simulink library "ammclib_bam_s32k14x"  (Simulink 9.0)
settings: Solver=ode45  StartTime=0.0  StopTime=10.0  RelTol=1e-3
undefined symbols (not defined in the file): f16A1, f16A2, f16B0, f16B1, f16B2, f16C1, f16CC1, f16CC1sc, f16CC1sc_D, f16CC1sc_Q, f16CC1scD, f16CC1scQ, f16CC2, f16CC2sc, f16CC2sc_D, f16CC2sc_Q, f16CC2scD, f16CC2scQ, f16DerivGain, f16EGain, f16FiltCoef, f16HystOff, f16HystOn, f16IGain, f16IntegGain, f16IntegGainFW, f16IntegGainQ, f16Kd, f16Kq, f16Limit, f16LowerLim, f16LowerLimit_D, f16LowerLimit_Q, f16ModIndex, f16OutValOff, f16OutValOn, f16PropGain, f16PropGainFW, f16PropGainQ, f16RampDown, f16RampUp, f16UGain, f16UpperLim, f16UpperLimit, f16UpperLimit_D, f16UpperLimit_Q, f16WIGain, f32A1, f32A2, f32B0, f32B1, f32B2, f32C1, f32CC1, f32CC1sc, f32CC1sc_D, f32CC1sc_Q, f32CC1scD, f32CC1scQ, f32CC2 ... (+122)
(part 6 of 11)

== system ammclib_bam_s32k14x/GFLIB/bam_f16/GFLIB_ControllerPIDpAW_F16 ==
  note: ---------------------------------------------------------------------------------------------------------------------------------------------------------------------------------------------------
  f16InErr : Inport
  f16UpperLimit : Inport  Port=2
  f16LowerLimit : Inport  Port=3
  GFLIB_ControllerPIDpAW_SF : S-Function  FunctionName=GFLIB_ControllerPIDpAW_SF_F16  Parameters=f16PropGain,s16PropGainShift,f16IntegGain,s16IntegGainShift,f16DerivGain,s16DerivGainShift,f16FiltCoef  SFunctionDeploymentMode=off  EnableBusSupport=off
  Unit_Delay_f16DerivPartK_1 : Delay  DelayLength=1  InitialCondition=0
  Unit_Delay_f16InK_1 : Delay  DelayLength=1  InitialCondition=0
  Unit_Delay_f32IntegPartK_1 : Delay  DelayLength=1  InitialCondition=0
  copyright : Subsystem
      mask Display: text(10,90,'FILE:');text(10,75,'DESRIPTION:');text(10,60,'COPYRIGHT:');text(10,45,'VERSION:');text(10,30,'DATE:')
  copyright2 : Subsystem
      mask Display: text(10,90,'GFLIB_ControllerPIDpAW_BAM_F16.mdl');text(10,75,'Parallel form of a standard PID controller with implemented anti-windup.');text(10,60,'NXP');text(10,45,'0.1');text(10,30,'21-Nov-2018');
  logo : Subsystem
      mask Display: image(imread('logo.jpg'))
  f16Out : Outport
  u16LimitFlag : Outport  Port=2
  wires:
  f16InErr/1 -> GFLIB_ControllerPIDpAW_SF/1
  f16UpperLimit/1 -> GFLIB_ControllerPIDpAW_SF/2
  f16LowerLimit/1 -> GFLIB_ControllerPIDpAW_SF/3
  Unit_Delay_f16InK_1/1 -> GFLIB_ControllerPIDpAW_SF/4
  Unit_Delay_f32IntegPartK_1/1 -> GFLIB_ControllerPIDpAW_SF/5
  Unit_Delay_f16DerivPartK_1/1 -> GFLIB_ControllerPIDpAW_SF/6
  GFLIB_ControllerPIDpAW_SF/1 -> f16Out/1
  GFLIB_ControllerPIDpAW_SF/2 -> u16LimitFlag/1
  GFLIB_ControllerPIDpAW_SF/3 -> Unit_Delay_f16InK_1/1
  GFLIB_ControllerPIDpAW_SF/4 -> Unit_Delay_f32IntegPartK_1/1
  GFLIB_ControllerPIDpAW_SF/5 -> Unit_Delay_f16DerivPartK_1/1

== system ammclib_bam_s32k14x/GFLIB/bam_f16/GFLIB_ControllerPIpAW_F16 ==
  note: ---------------------------------------------------------------------------------------------------------------------------------------------------------------------------------------------------
  f16InErr : Inport
  f16UpperLimit : Inport  Port=2
  f16LowerLimit : Inport  Port=3
  GFLIB_ControllerPIpAW_SF : S-Function  FunctionName=GFLIB_ControllerPIpAW_SF_F16  Parameters=f16PropGain,s16PropGainShift,f16IntegGain,s16IntegGainShift  SFunctionDeploymentMode=off  EnableBusSupport=off
  Unit_Delay_f16InK_1 : Delay  DelayLength=1  InitialCondition=0
  Unit_Delay_f32IntegPartK_1 : Delay  DelayLength=1  InitialCondition=0
  copyright : Subsystem
      mask Display: text(10,90,'FILE:');text(10,75,'DESRIPTION:');text(10,60,'COPYRIGHT:');text(10,45,'VERSION:');text(10,30,'DATE:')
  copyright2 : Subsystem
      mask Display: text(10,90,'GFLIB_ControllerPIpAW_BAM_F16.mdl');text(10,75,'Parallel form of a standard PI controller with implemented anti-windup.');text(10,60,'NXP');text(10,45,'0.1');text(10,30,'12-Jun-2015');
  logo : Subsystem
      mask Display: image(imread('logo.jpg'))
  f16Out : Outport
  u16LimitFlag : Outport  Port=2
  wires:
  GFLIB_ControllerPIpAW_SF/2 -> u16LimitFlag/1
  GFLIB_ControllerPIpAW_SF/1 -> f16Out/1
  f16LowerLimit/1 -> GFLIB_ControllerPIpAW_SF/3
  f16UpperLimit/1 -> GFLIB_ControllerPIpAW_SF/2
  f16InErr/1 -> GFLIB_ControllerPIpAW_SF/1
  Unit_Delay_f32IntegPartK_1/1 -> GFLIB_ControllerPIpAW_SF/5
  Unit_Delay_f16InK_1/1 -> GFLIB_ControllerPIpAW_SF/4
  GFLIB_ControllerPIpAW_SF/4 -> Unit_Delay_f32IntegPartK_1/1
  GFLIB_ControllerPIpAW_SF/3 -> Unit_Delay_f16InK_1/1

== system ammclib_bam_s32k14x/GFLIB/bam_f16/GFLIB_ControllerPIp_F16 ==
  note: ---------------------------------------------------------------------------------------------------------------------------------------------------------------------------------------------------
  f16InErr : Inport
  GFLIB_ControllerPIp_SF : S-Function  FunctionName=GFLIB_ControllerPIp_SF_F16  Parameters=f16PropGain,s16PropGainShift,f16IntegGain,s16IntegGainShift  SFunctionDeploymentMode=off  EnableBusSupport=off
  Unit_Delay_f32InIntegPartK_1 : UnitDelay  SampleTime=-1
  Unit_Delay_f32InK_1 : UnitDelay  SampleTime=-1
  copyright : Subsystem
      mask Display:
      | text(10,90,'FILE:');text(10,75,'DESRIPTION:')
      | text(10,60,'COPYRIGHT:')
      | text(10,45,'VERSION:')
      | text(10,30,'DATE:')
  copyright2 : Subsystem
      mask Display:
      | text(10,90,'GFLIB_ControllerPIp_BAM_F16.mdl');text(10,75,'Parallel form of a standard PI controller without implemented anti-windup.');text(10,60,'NXP')
      | text(10,45,'0.1');text(10,30,'20-Jan-2012');
  logo : Subsystem
      mask Display: image(imread('logo.jpg'))
  f16Out : Outport
  wires:
  GFLIB_ControllerPIp_SF/1 -> f16Out/1
  f16InErr/1 -> GFLIB_ControllerPIp_SF/1
  GFLIB_ControllerPIp_SF/3 -> Unit_Delay_f32InIntegPartK_1/1
  GFLIB_ControllerPIp_SF/2 -> Unit_Delay_f32InK_1/1
  Unit_Delay_f32InIntegPartK_1/1 -> GFLIB_ControllerPIp_SF/3
  Unit_Delay_f32InK_1/1 -> GFLIB_ControllerPIp_SF/2

== system ammclib_bam_s32k14x/GFLIB/bam_f16/GFLIB_ControllerPIrAW_F16 ==
  note: ---------------------------------------------------------------------------------------------------------------------------------------------------------------------------------------------------
  f16InErr : Inport
  f16UpperLimit : Inport  Port=2
  f16LowerLimit : Inport  Port=3
  GFLIB_ControllerPIrAW_SF : S-Function  FunctionName=GFLIB_ControllerPIrAW_SF_F16  Parameters=f16CC1,f16CC2,u16NShift  SFunctionDeploymentMode=off  EnableBusSupport=off
  Unit_Delay_f16InErrK1 : Delay  DelayLength=1  InitialCondition=0
  Unit_Delay_f32Acc : Delay  DelayLength=1  InitialCondition=0
  copyright : Subsystem
      mask Display: text(10,90,'FILE:');text(10,75,'DESRIPTION:');text(10,60,'COPYRIGHT:');text(10,45,'VERSION:');text(10,30,'DATE:')
  copyright2 : Subsystem
      mask Display: text(10,90,'GFLIB_ControllerPIrAW_BAM_F16.mdl');text(10,75,'Recurrent form of a standard PI controller with implemented anti-windup functionality.');text(10,60,'NXP');text(10,45,'0.1');text(10,30,'12-Jun-2015');
  logo : Subsystem
      mask Display: image(imread('logo.jpg'))
  f16Out : Outport
  wires:
  GFLIB_ControllerPIrAW_SF/3 -> Unit_Delay_f16InErrK1/1
  GFLIB_ControllerPIrAW_SF/2 -> Unit_Delay_f32Acc/1
  GFLIB_ControllerPIrAW_SF/1 -> f16Out/1
  f16LowerLimit/1 -> GFLIB_ControllerPIrAW_SF/3
  f16UpperLimit/1 -> GFLIB_ControllerPIrAW_SF/2
  f16InErr/1 -> GFLIB_ControllerPIrAW_SF/1
  Unit_Delay_f16InErrK1/1 -> GFLIB_ControllerPIrAW_SF/5
  Unit_Delay_f32Acc/1 -> GFLIB_ControllerPIrAW_SF/4

== system ammclib_bam_s32k14x/GFLIB/bam_f16/GFLIB_ControllerPIr_F16 ==
  note: ---------------------------------------------------------------------------------------------------------------------------------------------------------------------------------------------------
  f16InErr : Inport
  GFLIB_ControllerPIr_SF : S-Function  FunctionName=GFLIB_ControllerPIr_SF_F16  Parameters=f16CC1,f16CC2,u16NShift  SFunctionDeploymentMode=off  EnableBusSupport=off
  Unit_Delay_f16InErrK_1 : UnitDelay  SampleTime=-1
  Unit_Delay_f32AccIn : UnitDelay  SampleTime=-1
  copyright : Subsystem
      mask Display:
      | text(10,90,'FILE:');text(10,75,'DESRIPTION:')
      | text(10,60,'COPYRIGHT:')
      | text(10,45,'VERSION:')
      | text(10,30,'DATE:')
  copyright2 : Subsystem
      mask Display:
      | text(10,90,'GFLIB_ControllerPIr_BAM_F16.mdl');text(10,75,'Recurrent form of a standard PI controller without implemented anti-windup.');text(10,60,'NXP')
      | text(10,45,'0.1');text(10,30,'20-Jan-2012');
  logo : Subsystem
      mask Display: image(imread('logo.jpg'))
  f16Out : Outport
  wires:
  GFLIB_ControllerPIr_SF/1 -> f16Out/1
  f16InErr/1 -> GFLIB_ControllerPIr_SF/1
  GFLIB_ControllerPIr_SF/3 -> Unit_Delay_f16InErrK_1/1
  GFLIB_ControllerPIr_SF/2 -> Unit_Delay_f32AccIn/1
  Unit_Delay_f16InErrK_1/1 -> GFLIB_ControllerPIr_SF/3
  Unit_Delay_f32AccIn/1 -> GFLIB_ControllerPIr_SF/2

== system ammclib_bam_s32k14x/GFLIB/bam_f16/GFLIB_Cos_F16 ==
  note: ---------------------------------------------------------------------------------------------------------------------------------------------------------------------------------------------------
  f16In : Inport
  GFLIB_Cos_SF : S-Function  FunctionName=GFLIB_Cos_SF_F16  SFunctionDeploymentMode=off  EnableBusSupport=off
  copyright : Subsystem
      mask Display:
      | text(10,90,'FILE:');text(10,75,'DESRIPTION:')
      | text(10,60,'COPYRIGHT:')
      | text(10,45,'VERSION:')
      | text(10,30,'DATE:')
  copyright2 : Subsystem
      mask Display:
      | text(10,90,'GFLIB_Cos_BAM_F16.mdl');text(10,75,'Cosine transformation');text(10,60,'NXP')
      | text(10,45,'0.1');text(10,30,'13-Sep-2011');
  logo : Subsystem
      mask Display: image(imread('logo.jpg'))
  f16Out : Outport
  wires:
  GFLIB_Cos_SF/1 -> f16Out/1
  f16In/1 -> GFLIB_Cos_SF/1

== system ammclib_bam_s32k14x/GFLIB/bam_f16/GFLIB_Hyst_F16 ==
  note: ---------------------------------------------------------------------------------------------------------------------------------------------------------------------------------------------------
  f16In : Inport
  GFLIB_Hyst_SF_F16 : S-Function  FunctionName=GFLIB_Hyst_SF_F16  Parameters=f16HystOn,f16HystOff,f16OutValOn,f16OutValOff  SFunctionDeploymentMode=off  EnableBusSupport=off
  Unit_Delay_f16InState : UnitDelay  SampleTime=-1
  copyright : Subsystem
      mask Display:
      | text(10,90,'FILE:');text(10,75,'DESRIPTION:')
      | text(10,60,'COPYRIGHT:')
      | text(10,45,'VERSION:')
      | text(10,30,'DATE:')
  copyright2 : Subsystem
      mask Display:
      | text(10,90,'GFLIB_Hyst_BAM_F16.mdl');text(10,75,'Hysteresis function.');text(10,60,'NXP')
      | text(10,45,'0.1');text(10,30,'09-Apr-2014');
  logo : Subsystem
      mask Display: image(imread('logo.jpg'))
  f16Out : Outport
  wires:
  GFLIB_Hyst_SF_F16/1 -> f16Out/1
  f16In/1 -> GFLIB_Hyst_SF_F16/1
  Unit_Delay_f16InState/1 -> GFLIB_Hyst_SF_F16/2
  GFLIB_Hyst_SF_F16/2 -> Unit_Delay_f16InState/1

== system ammclib_bam_s32k14x/GFLIB/bam_f16/GFLIB_IntegratorTR_F16 ==
  note: ---------------------------------------------------------------------------------------------------------------------------------------------------------------------------------------------------
  f16In : Inport
  GFLIB_IntegratorTR_SF : S-Function  FunctionName=GFLIB_IntegratorTR_SF_F16  Parameters=f16C1,u16NShift  SFunctionDeploymentMode=off  EnableBusSupport=off
  Unit_Delay_f16InK_1 : UnitDelay  SampleTime=-1
  Unit_Delay_f32InAcc : UnitDelay  SampleTime=-1
  copyright : Subsystem
      mask Display:
      | text(10,90,'FILE:');text(10,75,'DESRIPTION:')
      | text(10,60,'COPYRIGHT:')
      | text(10,45,'VERSION:')
      | text(10,30,'DATE:')
  copyright2 : Subsystem
      mask Display:
      | text(10,90,'GFLIB_IntegratorTR_BAM_F16.mdl');text(10,75,'Discrete integrator transformed from linear model using Billinear (trapezoidal) transformation.');text(10,60,'NXP')
      | text(10,45,'0.1');text(10,30,'16-Jan-2012');
  logo : Subsystem
      mask Display: image(imread('logo.jpg'))
  f16Out : Outport
  wires:
  GFLIB_IntegratorTR_SF/1 -> f16Out/1
  f16In/1 -> GFLIB_IntegratorTR_SF/1
  Unit_Delay_f16InK_1/1 -> GFLIB_IntegratorTR_SF/3
  GFLIB_IntegratorTR_SF/3 -> Unit_Delay_f16InK_1/1
  Unit_Delay_f32InAcc/1 -> GFLIB_IntegratorTR_SF/2
  GFLIB_IntegratorTR_SF/2 -> Unit_Delay_f32InAcc/1

== system ammclib_bam_s32k14x/GFLIB/bam_f16/GFLIB_Limit_F16 ==
  note: ---------------------------------------------------------------------------------------------------------------------------------------------------------------------------------------------------
  f16In : Inport
  GFLIB_Limit_SF_F16 : S-Function  FunctionName=GFLIB_Limit_SF_F16  Parameters=f16UpperLimit,f16LowerLim  SFunctionDeploymentMode=off  EnableBusSupport=off
  copyright : Subsystem
      mask Display:
      | text(10,90,'FILE:');text(10,75,'DESRIPTION:')
      | text(10,60,'COPYRIGHT:')
      | text(10,45,'VERSION:')
      | text(10,30,'DATE:')
      | text(10,15,'AUTHOR:')
  copyright2 : Subsystem
      mask Display:
      | text(10,90,'GFLIB_Limit_BAM_F16.mdl');text(10,75,'Limit function');text(10,60,'NXP')
      | text(10,45,'0.1');text(10,30,'03-Jul-2011');text(10,15,'');
  logo : Subsystem
      mask Display: image(imread('logo.jpg'))
  f16Out : Outport
  wires:
  GFLIB_Limit_SF_F16/1 -> f16Out/1
  f16In/1 -> GFLIB_Limit_SF_F16/1

== system ammclib_bam_s32k14x/GFLIB/bam_f16/GFLIB_LowerLimit_F16 ==
  note: ---------------------------------------------------------------------------------------------------------------------------------------------------------------------------------------------------
  f16In : Inport
  GFLIB_LowerLimit_SF_F16 : S-Function  FunctionName=GFLIB_LowerLimit_SF_F16  Parameters=f16LowerLim  SFunctionDeploymentMode=off  EnableBusSupport=off
  copyright : Subsystem
      mask Display:
      | text(10,90,'FILE:');text(10,75,'DESRIPTION:')
      | text(10,60,'COPYRIGHT:')
      | text(10,45,'VERSION:')
      | text(10,30,'DATE:')
  copyright2 : Subsystem
      mask Display:
      | text(10,90,'GFLIB_LowerLimit_BAM_F16.mdl');text(10,75,'Lower limit function.');text(10,60,'Freescale')
      | text(10,45,'0.1');text(10,30,'13-Sep-2011');
  logo : Subsystem
      mask Display: image(imread('logo.jpg'))
  f16Out : Outport
  wires:
  GFLIB_LowerLimit_SF_F16/1 -> f16Out/1
  f16In/1 -> GFLIB_LowerLimit_SF_F16/1

== system ammclib_bam_s32k14x/GFLIB/bam_f16/GFLIB_Lut1D_F16 ==
  note: ---------------------------------------------------------------------------------------------------------------------------------------------------------------------------------------------------
  f16In : Inport
  GFLIB_Lut1D_SF : S-Function  FunctionName=GFLIB_Lut1D_SF_F16  Parameters=u16ShamOffset,pf16Table,s16MidIdx  SFunctionDeploymentMode=off  EnableBusSupport=off
  copyright : Subsystem
      mask Display:
      | text(10,90,'FILE:');text(10,75,'DESRIPTION:')
      | text(10,60,'COPYRIGHT:')
      | text(10,45,'VERSION:')
      | text(10,30,'DATE:')
  copyright2 : Subsystem
      mask Display:
      | text(10,90,'GFLIB_Lut1D_BAM_F16.mdl');text(10,75,'One dimensional Look-up table function');text(10,60,'NXP')
      | text(10,45,'0.1');text(10,30,'17-Jun-2013');
  logo : Subsystem
      mask Display: image(imread('logo.jpg'))
  f16Out : Outport
  wires:
  GFLIB_Lut1D_SF/1 -> f16Out/1
  f16In/1 -> GFLIB_Lut1D_SF/1

== system ammclib_bam_s32k14x/GFLIB/bam_f16/GFLIB_Lut2D_F16 ==
  note: ---------------------------------------------------------------------------------------------------------------------------------------------------------------------------------------------------
  f16In1 : Inport
  f16In2 : Inport  Port=2
  GFLIB_Lut2D_SF : S-Function  FunctionName=GFLIB_Lut2D_SF_F16  Parameters=u16ShamOffset1,u16ShamOffset2,pf16Table,s16MidIdx  SFunctionDeploymentMode=off  EnableBusSupport=off
  copyright : Subsystem
      mask Display:
      | text(10,90,'FILE:');text(10,75,'DESRIPTION:')
      | text(10,60,'COPYRIGHT:')
      | text(10,45,'VERSION:')
      | text(10,30,'DATE:')
  copyright2 : Subsystem
      mask Display:
      | text(10,90,'GFLIB_Lut2D_BAM_F16.mdl');text(10,75,'Two dimensional Look-up table function');text(10,60,'NXP')
      | text(10,45,'0.1');text(10,30,'17-Jun-2013');
  logo : Subsystem
      mask Display: image(imread('logo.jpg'))
  f16Out : Outport
  wires:
  GFLIB_Lut2D_SF/1 -> f16Out/1
  f16In2/1 -> GFLIB_Lut2D_SF/2
  f16In1/1 -> GFLIB_Lut2D_SF/1

== system ammclib_bam_s32k14x/GFLIB/bam_f16/GFLIB_Ramp_F16 ==
  note: ---------------------------------------------------------------------------------------------------------------------------------------------------------------------------------------------------
  f16In : Inport
  GFLIB_Ramp_SF_F16 : S-Function  FunctionName=GFLIB_Ramp_SF_F16  Parameters=f16RampUp,f16RampDown  SFunctionDeploymentMode=off  EnableBusSupport=off
  Unit_Delay_f16InState : UnitDelay  SampleTime=-1
  copyright : Subsystem
      mask Display:
      | text(10,90,'FILE:');text(10,75,'DESRIPTION:')
      | text(10,60,'COPYRIGHT:')
      | text(10,45,'VERSION:')
      | text(10,30,'DATE:')
      | text(10,15,'AUTHOR:')
  copyright2 : Subsystem
      mask Display:
      | text(10,90,'GFLIB_Ramp_BAM_F16.mdl');text(10,75,'Rate of change limiter - Ramp function.');text(10,60,'NXP')
      | text(10,45,'0.1');text(10,30,'08-Apr-2014');text(10,15,'');
  logo : Subsystem
      mask Display: image(imread('logo.jpg'))
  f16Out : Outport
  wires:
  GFLIB_Ramp_SF_F16/1 -> f16Out/1
  f16In/1 -> GFLIB_Ramp_SF_F16/1
  Unit_Delay_f16InState/1 -> GFLIB_Ramp_SF_F16/2
  GFLIB_Ramp_SF_F16/2 -> Unit_Delay_f16InState/1

== system ammclib_bam_s32k14x/GFLIB/bam_f16/GFLIB_Sign_F16 ==
  note: ---------------------------------------------------------------------------------------------------------------------------------------------------------------------------------------------------
  f16In : Inport
  GFLIB_Sign_SF_F16 : S-Function  FunctionName=GFLIB_Sign_SF_F16  SFunctionDeploymentMode=off  EnableBusSupport=off
  copyright : Subsystem
      mask Display:
      | text(10,90,'FILE:');text(10,75,'DESRIPTION:')
      | text(10,60,'COPYRIGHT:')
      | text(10,45,'VERSION:')
      | text(10,30,'DATE:')
  copyright2 : Subsystem
      mask Display:
      | text(10,90,'GFLIB_Sign_BAM_F16.mdl');text(10,75,'Sign function.');text(10,60,'NXP')
      | text(10,45,'0.1');text(10,30,'26-Aug-2011');
  logo : Subsystem
      mask Display: image(imread('logo.jpg'))
  f16Out : Outport
  wires:
  GFLIB_Sign_SF_F16/1 -> f16Out/1
  f16In/1 -> GFLIB_Sign_SF_F16/1

== system ammclib_bam_s32k14x/GFLIB/bam_f16/GFLIB_SinCos_F16 ==
  note: ---------------------------------------------------------------------------------------------------------------------------------------------------------------------------------------------------
  f16In : Inport
  GFLIB_SinCos_SF : S-Function  FunctionName=GFLIB_SinCos_SF_F16  SFunctionDeploymentMode=off  EnableBusSupport=off
  copyright : Subsystem
      mask Display: text(10,90,'FILE:');text(10,75,'DESRIPTION:');text(10,60,'COPYRIGHT:');text(10,45,'VERSION:');text(10,30,'DATE:')
  copyright2 : Subsystem
      mask Display: text(10,90,'GFLIB_SinCos_BAM_F16.mdl');text(10,75,'Sine and Cosine transformation');text(10,60,'Freescale');text(10,45,'0.1');text(10,30,'27-Sep-2015');
  logo : Subsystem
      mask Display: image(imread('logo.jpg'))
  f16SinOut : Outport
  f16CosOut : Outport  Port=2
  wires:
  GFLIB_SinCos_SF/2 -> f16CosOut/1
  GFLIB_SinCos_SF/1 -> f16SinOut/1
  f16In/1 -> GFLIB_SinCos_SF/1

== system ammclib_bam_s32k14x/GFLIB/bam_f16/GFLIB_Sin_F16 ==
  note: ---------------------------------------------------------------------------------------------------------------------------------------------------------------------------------------------------
  f16In : Inport
  GFLIB_Sin_SF : S-Function  FunctionName=GFLIB_Sin_SF_F16  SFunctionDeploymentMode=off  EnableBusSupport=off
  copyright : Subsystem
      mask Display:
      | text(10,90,'FILE:');text(10,75,'DESRIPTION:')
      | text(10,60,'COPYRIGHT:')
      | text(10,45,'VERSION:')
      | text(10,30,'DATE:')
  copyright2 : Subsystem
      mask Display:
      | text(10,90,'GFLIB_Sin_BAM_F16.mdl');text(10,75,'Sine transformation');text(10,60,'NXP')
      | text(10,45,'0.1');text(10,30,'13-Sep-2011');
  logo : Subsystem
      mask Display: image(imread('logo.jpg'))
  f16Out : Outport
  wires:
  GFLIB_Sin_SF/1 -> f16Out/1
  f16In/1 -> GFLIB_Sin_SF/1

== system ammclib_bam_s32k14x/GFLIB/bam_f16/GFLIB_Sqrt_F16 ==
  note: ---------------------------------------------------------------------------------------------------------------------------------------------------------------------------------------------------
  f16In : Inport
  GFLIB_Sqrt_SF_F16 : S-Function  FunctionName=GFLIB_Sqrt_SF_F16  SFunctionDeploymentMode=off  EnableBusSupport=off
  copyright : Subsystem
      mask Display:
      | text(10,90,'FILE:');text(10,75,'DESRIPTION:')
      | text(10,60,'COPYRIGHT:')
      | text(10,45,'VERSION:')
      | text(10,30,'DATE:')
  copyright2 : Subsystem
      mask Display:
      | text(10,90,'GFLIB_Sqrt_BAM_F16.mdl');text(10,75,'Square root approximation.');text(10,60,'Freescale')
      | text(10,45,'0.1');text(10,30,'12-Sep-2011');
  logo : Subsystem
      mask Display: image(imread('logo.jpg'))
  f16Out : Outport
  wires:
  GFLIB_Sqrt_SF_F16/1 -> f16Out/1
  f16In/1 -> GFLIB_Sqrt_SF_F16/1

== system ammclib_bam_s32k14x/GFLIB/bam_f16/GFLIB_Tan_F16 ==
  note: ---------------------------------------------------------------------------------------------------------------------------------------------------------------------------------------------------
  f16In : Inport
  GFLIB_Tan_SF : S-Function  FunctionName=GFLIB_Tan_SF_F16  SFunctionDeploymentMode=off  EnableBusSupport=off
  copyright : Subsystem
      mask Display:
      | text(10,90,'FILE:');text(10,75,'DESRIPTION:')
      | text(10,60,'COPYRIGHT:')
      | text(10,45,'VERSION:')
      | text(10,30,'DATE:')
  copyright2 : Subsystem
      mask Display:
      | text(10,90,'GFLIB_Tan_BAM_F16.mdl');text(10,75,'Tangent transformation');text(10,60,'NXP')
      | text(10,45,'0.1');text(10,30,'13-Sep-2011');
  logo : Subsystem
      mask Display: image(imread('logo.jpg'))
  f16Out : Outport
  wires:
  GFLIB_Tan_SF/1 -> f16Out/1
  f16In/1 -> GFLIB_Tan_SF/1

== system ammclib_bam_s32k14x/GFLIB/bam_f16/GFLIB_UpperLimit_F16 ==
  note: ---------------------------------------------------------------------------------------------------------------------------------------------------------------------------------------------------
  f16In : Inport
  GFLIB_UpperLimit_SF_F16 : S-Function  FunctionName=GFLIB_UpperLimit_SF_F16  Parameters=f16UpperLim  SFunctionDeploymentMode=off  EnableBusSupport=off
  copyright : Subsystem
      mask Display:
      | text(10,90,'FILE:');text(10,75,'DESRIPTION:')
      | text(10,60,'COPYRIGHT:')
      | text(10,45,'VERSION:')
      | text(10,30,'DATE:')
  copyright2 : Subsystem
      mask Display:
      | text(10,90,'GFLIB_UpperLimit_BAM_F16.mdl');text(10,75,'Upper limit function.');text(10,60,'Freescale')
      | text(10,45,'0.1');text(10,30,'13-Sep-2011');
  logo : Subsystem
      mask Display: image(imread('logo.jpg'))
  f16Out : Outport
  wires:
  GFLIB_UpperLimit_SF_F16/1 -> f16Out/1
  f16In/1 -> GFLIB_UpperLimit_SF_F16/1

== system ammclib_bam_s32k14x/GFLIB/bam_f16/GFLIB_VMin_F16 ==
  note: ---------------------------------------------------------------------------------------------------------------------------------------------------------------------------------------------------
  InputVector : Inport
  GFLIB_VMin_SF : S-Function  FunctionName=GFLIB_VMin_SF_F16  Parameters=N  SFunctionDeploymentMode=off  EnableBusSupport=off
  Gain : Gain  Gain=[eye(N) zeros(N,256-N)]'  Multiplication=Matrix(K*u)  OutDataTypeStr=int16
  copyright : Subsystem
      mask Display: text(10,90,'FILE:');text(10,75,'DESRIPTION:');text(10,60,'COPYRIGHT:');text(10,45,'VERSION:');text(10,30,'DATE:')
  copyright2 : Subsystem
      mask Display: text(10,90,'GFLIB_VMin_BAM_F16.mdl');text(10,75,'Vector minimum');text(10,60,'NXP');text(10,45,'1.0');text(10,30,'18-Jan-2018');
  logo : Subsystem
      mask Display: image(imread('logo.jpg'))
  IndexOfMinimum : Outport
  wires:
  InputVector/1 -> Gain/1
  GFLIB_VMin_SF/1 -> IndexOfMinimum/1
  Gain/1 -> GFLIB_VMin_SF/1

== system ammclib_bam_s32k14x/GFLIB/bam_f16/GFLIB_VectorLimit_F16 ==
  note: ---------------------------------------------------------------------------------------------------------------------------------------------------------------------------------------------------
  f16InVec1 : Inport
  f16InVec2 : Inport  Port=2
  GFLIB_VectorLimit_SF_F16 : S-Function  FunctionName=GFLIB_VectorLimit_SF_F16  Parameters=f16Limit  SFunctionDeploymentMode=off  EnableBusSupport=off
  copyright : Subsystem
      mask Display:
      | text(10,90,'FILE:');text(10,75,'DESRIPTION:')
      | text(10,60,'COPYRIGHT:')
      | text(10,45,'VERSION:')
      | text(10,30,'DATE:')
      | text(10,15,'AUTHOR:')
  copyright2 : Subsystem
      mask Display:
      | text(10,90,'GFLIB_VectorLimit_BAM_F16.mdl');text(10,75,'Vector limit function');text(10,60,'Freescale')
      | text(10,45,'0.1');text(10,30,'15-Sep-2011');text(10,15,'');
  logo : Subsystem
      mask Display: image(imread('logo.jpg'))
  f16OutVec1 : Outport
  f16OutVec2 : Outport  Port=2
  bFlag : Outport  Port=3
  wires:
  GFLIB_VectorLimit_SF_F16/3 -> bFlag/1
  GFLIB_VectorLimit_SF_F16/2 -> f16OutVec2/1
  f16InVec2/1 -> GFLIB_VectorLimit_SF_F16/2
  GFLIB_VectorLimit_SF_F16/1 -> f16OutVec1/1
  f16InVec1/1 -> GFLIB_VectorLimit_SF_F16/1

== system ammclib_bam_s32k14x/GFLIB/bam_f32/GFLIB_Acos_F32 ==
  note: ---------------------------------------------------------------------------------------------------------------------------------------------------------------------------------------------------
  f32In : Inport
  GFLIB_Acos_SF : S-Function  FunctionName=GFLIB_Acos_SF_F32  SFunctionDeploymentMode=off  EnableBusSupport=off
  copyright : Subsystem
      mask Display:
      | text(10,90,'FILE:');text(10,75,'DESRIPTION:')
      | text(10,60,'COPYRIGHT:')
      | text(10,45,'VERSION:')
      | text(10,30,'DATE:')
  copyright2 : Subsystem
      mask Display:
      | text(10,90,'GFLIB_Acos_BAM_F32.mdl');text(10,75,'Inverse cosine transformation');text(10,60,'Freescale')
      | text(10,45,'0.1');text(10,30,'31-Aug-2011');
  logo : Subsystem
      mask Display: image(imread('logo.jpg'))
  f32Out : Outport
  wires:
  GFLIB_Acos_SF/1 -> f32Out/1
  f32In/1 -> GFLIB_Acos_SF/1

== system ammclib_bam_s32k14x/GFLIB/bam_f32/GFLIB_Asin_F32 ==
  note: ---------------------------------------------------------------------------------------------------------------------------------------------------------------------------------------------------
  f32In : Inport
  GFLIB_Asin_SF : S-Function  FunctionName=GFLIB_Asin_SF_F32  SFunctionDeploymentMode=off  EnableBusSupport=off
  copyright : Subsystem
      mask Display:
      | text(10,90,'FILE:');text(10,75,'DESRIPTION:')
      | text(10,60,'COPYRIGHT:')
      | text(10,45,'VERSION:')
      | text(10,30,'DATE:')
  copyright2 : Subsystem
      mask Display:
      | text(10,90,'GFLIB_Asin_BAM_F32.mdl');text(10,75,'Inverse cosine transformation');text(10,60,'Freescale')
      | text(10,45,'0.1');text(10,30,'01-Sep-2011');
  logo : Subsystem
      mask Display: image(imread('logo.jpg'))
  f32Out : Outport
  wires:
  GFLIB_Asin_SF/1 -> f32Out/1
  f32In/1 -> GFLIB_Asin_SF/1

== system ammclib_bam_s32k14x/GFLIB/bam_f32/GFLIB_AtanYXShifted_F32 ==
  note: ---------------------------------------------------------------------------------------------------------------------------------------------------------------------------------------------------
  f32InY : Inport
  f32InX : Inport  Port=2
  GFLIB_AtanYXShifted_SF : S-Function  FunctionName=GFLIB_AtanYXShifted_SF_F32  Parameters=Ky,Kx,Ny,Nx,ThetaAdj  SFunctionDeploymentMode=off  EnableBusSupport=off
  copyright : Subsystem
      mask Display:
      | text(10,90,'FILE:');text(10,75,'DESRIPTION:')
      | text(10,60,'COPYRIGHT:')
      | text(10,45,'VERSION:')
      | text(10,30,'DATE:')
  copyright2 : Subsystem
      mask Display:
      | text(10,90,'GFLIB_AtanYXShifted_BAM_F32.mdl');text(10,75,'Shifted YX Arctangent of argument.');text(10,60,'NXP')
      | text(10,45,'0.1');text(10,30,'06-Sep-2011');
  logo : Subsystem
      mask Display: image(imread('logo.jpg'))
  f32Out : Outport
  wires:
  GFLIB_AtanYXShifted_SF/1 -> f32Out/1
  f32InX/1 -> GFLIB_AtanYXShifted_SF/2
  f32InY/1 -> GFLIB_AtanYXShifted_SF/1

== system ammclib_bam_s32k14x/GFLIB/bam_f32/GFLIB_AtanYX_F32 ==
  note: ---------------------------------------------------------------------------------------------------------------------------------------------------------------------------------------------------
  f32InY : Inport
  f32InX : Inport  Port=2
  GFLIB_AtanYX_SF : S-Function  FunctionName=GFLIB_AtanYX_SF_F32  SFunctionDeploymentMode=off  EnableBusSupport=off
  copyright : Subsystem
      mask Display:
      | text(10,90,'FILE:');text(10,75,'DESRIPTION:')
      | text(10,60,'COPYRIGHT:')
      | text(10,45,'VERSION:')
      | text(10,30,'DATE:')
  copyright2 : Subsystem
      mask Display:
      | text(10,90,'GFLIB_AtanYX_BAM_F32.mdl');text(10,75,'YX Arctangent of argument.');text(10,60,'Freescale')
      | text(10,45,'0.1');text(10,30,'05-Sep-2011');
  logo : Subsystem
      mask Display: image(imread('logo.jpg'))
  f32Out : Outport
  wires:
  GFLIB_AtanYX_SF/1 -> f32Out/1
  f32InX/1 -> GFLIB_AtanYX_SF/2
  f32InY/1 -> GFLIB_AtanYX_SF/1

== system ammclib_bam_s32k14x/GFLIB/bam_f32/GFLIB_Atan_F32 ==
  note: ---------------------------------------------------------------------------------------------------------------------------------------------------------------------------------------------------
  f32In : Inport
  GFLIB_Atan_SF : S-Function  FunctionName=GFLIB_Atan_SF_F32  SFunctionDeploymentMode=off  EnableBusSupport=off
  copyright : Subsystem
      mask Display:
      | text(10,90,'FILE:');text(10,75,'DESRIPTION:')
      | text(10,60,'COPYRIGHT:')
      | text(10,45,'VERSION:')
      | text(10,30,'DATE:')
  copyright2 : Subsystem
      mask Display:
      | text(10,90,'GFLIB_Atan_BAM_F32.mdl');text(10,75,'Inverse tangent transformation');text(10,60,'Freescale')
      | text(10,45,'0.1');text(10,30,'01-Sep-2011');
  logo : Subsystem
      mask Display: image(imread('logo.jpg'))
  f32Out : Outport
  wires:
  GFLIB_Atan_SF/1 -> f32Out/1
  f32In/1 -> GFLIB_Atan_SF/1

== system ammclib_bam_s32k14x/GFLIB/bam_f32/GFLIB_ControllerPIDpAW_F32 ==
  note: ---------------------------------------------------------------------------------------------------------------------------------------------------------------------------------------------------
  f32InErr : Inport
  f32UpperLimit : Inport  Port=2
  f32LowerLimit : Inport  Port=3
  Delay : Delay  DelayLength=1  InitialCondition=0
  Delay1 : Delay  DelayLength=1  InitialCondition=0
  Delay2 : Delay  DelayLength=1  InitialCondition=0
  GFLIB_ControllerPIDpAW_SF : S-Function  FunctionName=GFLIB_ControllerPIDpAW_SF_F32  Parameters=f32PropGain,s16PropGainShift,f32IntegGain,s16IntegGainShift,f32DerivGain,s16DerivGainShift,f32FiltCoef  SFunctionDeploymentMode=off  EnableBusSupport=off
  copyright : Subsystem
      mask Display: text(10,90,'FILE:');text(10,75,'DESRIPTION:');text(10,60,'COPYRIGHT:');text(10,45,'VERSION:');text(10,30,'DATE:')
  copyright2 : Subsystem
      mask Display: text(10,90,'GFLIB_ControllerPIDpAW_BAM_F32.mdl');text(10,75,'Parallel form of a standard PID controller with implemented anti-windup.');text(10,60,'NXP');text(10,45,'0.1');text(10,30,'21-Nov-2018');
  logo : Subsystem
      mask Display: image(imread('logo.jpg'))
  f32Out : Outport
  u16LimitFlag : Outport  Port=2
  wires:
  f32InErr/1 -> GFLIB_ControllerPIDpAW_SF/1
  f32UpperLimit/1 -> GFLIB_ControllerPIDpAW_SF/2
  f32LowerLimit/1 -> GFLIB_ControllerPIDpAW_SF/3
  Delay2/1 -> GFLIB_ControllerPIDpAW_SF/4
  Delay1/1 -> GFLIB_ControllerPIDpAW_SF/5
  Delay/1 -> GFLIB_ControllerPIDpAW_SF/6
  GFLIB_ControllerPIDpAW_SF/1 -> f32Out/1
  GFLIB_ControllerPIDpAW_SF/2 -> u16LimitFlag/1
  GFLIB_ControllerPIDpAW_SF/3 -> Delay2/1
  GFLIB_ControllerPIDpAW_SF/4 -> Delay1/1
  GFLIB_ControllerPIDpAW_SF/5 -> Delay/1

== system ammclib_bam_s32k14x/GFLIB/bam_f32/GFLIB_ControllerPIpAW_F32 ==
  note: ---------------------------------------------------------------------------------------------------------------------------------------------------------------------------------------------------
  f32InErr : Inport
  f32UpperLimit : Inport  Port=2
  f32LowerLimit : Inport  Port=3
  GFLIB_ControllerPIpAW_SF : S-Function  FunctionName=GFLIB_ControllerPIpAW_SF_F32  Parameters=f32PropGain,s16PropGainShift,f32IntegGain,s16IntegGainShift  SFunctionDeploymentMode=off  EnableBusSupport=off
  Unit_Delay_f32InK_1 : Delay  DelayLength=1  InitialCondition=0
  Unit_Delay_f32IntegPartK_1 : Delay  DelayLength=1  InitialCondition=0
  copyright : Subsystem
      mask Display: text(10,90,'FILE:');text(10,75,'DESRIPTION:');text(10,60,'COPYRIGHT:');text(10,45,'VERSION:');text(10,30,'DATE:')
  copyright2 : Subsystem
      mask Display: text(10,90,'GFLIB_ControllerPIpAW_BAM_F32.mdl');text(10,75,'Parallel form of a standard PI controller with implemented anti-windup.');text(10,60,'NXP');text(10,45,'0.1');text(10,30,'12-Jun-2015');
  logo : Subsystem
      mask Display: image(imread('logo.jpg'))
  f32Out : Outport
  u16LimitFlag : Outport  Port=2
  wires:
  GFLIB_ControllerPIpAW_SF/2 -> u16LimitFlag/1
  GFLIB_ControllerPIpAW_SF/1 -> f32Out/1
  f32LowerLimit/1 -> GFLIB_ControllerPIpAW_SF/3
  f32UpperLimit/1 -> GFLIB_ControllerPIpAW_SF/2
  f32InErr/1 -> GFLIB_ControllerPIpAW_SF/1
  Unit_Delay_f32IntegPartK_1/1 -> GFLIB_ControllerPIpAW_SF/5
  Unit_Delay_f32InK_1/1 -> GFLIB_ControllerPIpAW_SF/4
  GFLIB_ControllerPIpAW_SF/4 -> Unit_Delay_f32IntegPartK_1/1
  GFLIB_ControllerPIpAW_SF/3 -> Unit_Delay_f32InK_1/1

== system ammclib_bam_s32k14x/GFLIB/bam_f32/GFLIB_ControllerPIp_F32 ==
  note: ---------------------------------------------------------------------------------------------------------------------------------------------------------------------------------------------------
  f32InErr : Inport
  GFLIB_ControllerPIp_SF : S-Function  FunctionName=GFLIB_ControllerPIp_SF_F32  Parameters=f32PropGain,s16PropGainShift,f32IntegGain,s16IntegGainShift  SFunctionDeploymentMode=off  EnableBusSupport=off
  Unit_Delay_f32InIntegPartK_1 : UnitDelay  SampleTime=-1
  Unit_Delay_f32InK_1 : UnitDelay  SampleTime=-1
  copyright : Subsystem
      mask Display:
      | text(10,90,'FILE:');text(10,75,'DESRIPTION:')
      | text(10,60,'COPYRIGHT:')
      | text(10,45,'VERSION:')
      | text(10,30,'DATE:')
  copyright2 : Subsystem
      mask Display:
      | text(10,90,'GFLIB_ControllerPIp_BAM_F32.mdl');text(10,75,'Parallel form of a standard PI controller without implemented anti-windup.');text(10,60,'NXP')
      | text(10,45,'0.1');text(10,30,'20-Jan-2012');
  logo : Subsystem
      mask Display: image(imread('logo.jpg'))
  f32Out : Outport
  wires:
  GFLIB_ControllerPIp_SF/1 -> f32Out/1
  f32InErr/1 -> GFLIB_ControllerPIp_SF/1
  GFLIB_ControllerPIp_SF/3 -> Unit_Delay_f32InIntegPartK_1/1
  Unit_Delay_f32InIntegPartK_1/1 -> GFLIB_ControllerPIp_SF/3
  Unit_Delay_f32InK_1/1 -> GFLIB_ControllerPIp_SF/2
  GFLIB_ControllerPIp_SF/2 -> Unit_Delay_f32InK_1/1

== system ammclib_bam_s32k14x/GFLIB/bam_f32/GFLIB_ControllerPIrAW_F32 ==
  note: ---------------------------------------------------------------------------------------------------------------------------------------------------------------------------------------------------
  f32InErr : Inport
  f32UpperLimit : Inport  Port=2
  f32LowerLimit : Inport  Port=3
  GFLIB_ControllerPIrAW_SF : S-Function  FunctionName=GFLIB_ControllerPIrAW_SF_F32  Parameters=f32CC1,f32CC2,u16NShift  SFunctionDeploymentMode=off  EnableBusSupport=off
  Unit_Delay_f32Acc : Delay  DelayLength=1  InitialCondition=0
  Unit_Delay_f32InErrK1 : Delay  DelayLength=1  InitialCondition=0
  copyright : Subsystem
      mask Display: text(10,90,'FILE:');text(10,75,'DESRIPTION:');text(10,60,'COPYRIGHT:');text(10,45,'VERSION:');text(10,30,'DATE:')
  copyright2 : Subsystem
      mask Display: text(10,90,'GFLIB_ControllerPIrAW_BAM_F32.mdl');text(10,75,'Recurrent form of a standard PI controller with implemented anti-windup functionality.');text(10,60,'NXP');text(10,45,'0.1');text(10,30,'12-Jun-2015');
  logo : Subsystem
      mask Display: image(imread('logo.jpg'))
  f32Out : Outport
  wires:
  GFLIB_ControllerPIrAW_SF/1 -> f32Out/1
  f32LowerLimit/1 -> GFLIB_ControllerPIrAW_SF/3
  f32UpperLimit/1 -> GFLIB_ControllerPIrAW_SF/2
  f32InErr/1 -> GFLIB_ControllerPIrAW_SF/1
  GFLIB_ControllerPIrAW_SF/3 -> Unit_Delay_f32InErrK1/1
  GFLIB_ControllerPIrAW_SF/2 -> Unit_Delay_f32Acc/1
  Unit_Delay_f32InErrK1/1 -> GFLIB_ControllerPIrAW_SF/5
  Unit_Delay_f32Acc/1 -> GFLIB_ControllerPIrAW_SF/4

== system ammclib_bam_s32k14x/GFLIB/bam_f32/GFLIB_ControllerPIr_F32 ==
  note: ---------------------------------------------------------------------------------------------------------------------------------------------------------------------------------------------------
  f32InErr : Inport
  GFLIB_ControllerPIr_SF : S-Function  FunctionName=GFLIB_ControllerPIr_SF_F32  Parameters=f32CC1,f32CC2,u16NShift  SFunctionDeploymentMode=off  EnableBusSupport=off
  Unit_Delay_f32AccIn : UnitDelay  SampleTime=-1
  Unit_Delay_f32InErrK_1 : UnitDelay  SampleTime=-1
  copyright : Subsystem
      mask Display:
      | text(10,90,'FILE:');text(10,75,'DESRIPTION:')
      | text(10,60,'COPYRIGHT:')
      | text(10,45,'VERSION:')
      | text(10,30,'DATE:')
  copyright2 : Subsystem
      mask Display:
      | text(10,90,'GFLIB_ControllerPIr_BAM_F32.mdl');text(10,75,'Recurrent form of a standard PI controller without implemented anti-windup.');text(10,60,'NXP')
      | text(10,45,'0.1');text(10,30,'20-Jan-2012');
  logo : Subsystem
      mask Display: image(imread('logo.jpg'))
  f32Out : Outport
  wires:
  GFLIB_ControllerPIr_SF/1 -> f32Out/1
  f32InErr/1 -> GFLIB_ControllerPIr_SF/1
  Unit_Delay_f32InErrK_1/1 -> GFLIB_ControllerPIr_SF/3
  Unit_Delay_f32AccIn/1 -> GFLIB_ControllerPIr_SF/2
  GFLIB_ControllerPIr_SF/3 -> Unit_Delay_f32InErrK_1/1
  GFLIB_ControllerPIr_SF/2 -> Unit_Delay_f32AccIn/1

== system ammclib_bam_s32k14x/GFLIB/bam_f32/GFLIB_Cos_F32 ==
  note: ---------------------------------------------------------------------------------------------------------------------------------------------------------------------------------------------------
  f32In : Inport
  GFLIB_Cos_SF : S-Function  FunctionName=GFLIB_Cos_SF_F32  SFunctionDeploymentMode=off  EnableBusSupport=off
  copyright : Subsystem
      mask Display:
      | text(10,90,'FILE:');text(10,75,'DESRIPTION:')
      | text(10,60,'COPYRIGHT:')
      | text(10,45,'VERSION:')
      | text(10,30,'DATE:')
  copyright2 : Subsystem
      mask Display:
      | text(10,90,'GFLIB_Cos_BAM_F32.mdl');text(10,75,'Cosine transformation');text(10,60,'NXP')
      | text(10,45,'0.1');text(10,30,'13-Sep-2011');
  logo : Subsystem
      mask Display: image(imread('logo.jpg'))
  f32Out : Outport
  wires:
  GFLIB_Cos_SF/1 -> f32Out/1
  f32In/1 -> GFLIB_Cos_SF/1

== system ammclib_bam_s32k14x/GFLIB/bam_f32/GFLIB_Hyst_F32 ==
  note: ---------------------------------------------------------------------------------------------------------------------------------------------------------------------------------------------------
  f32In : Inport
  GFLIB_Hyst_SF_F32 : S-Function  FunctionName=GFLIB_Hyst_SF_F32  Parameters=f32HystOn,f32HystOff,f32OutValOn,f32OutValOff  SFunctionDeploymentMode=off  EnableBusSupport=off
  Unit_Delay_f32InState : UnitDelay  SampleTime=-1
  copyright : Subsystem
      mask Display:
      | text(10,90,'FILE:');text(10,75,'DESRIPTION:')
      | text(10,60,'COPYRIGHT:')
      | text(10,45,'VERSION:')
      | text(10,30,'DATE:')
  copyright2 : Subsystem
      mask Display:
      | text(10,90,'GFLIB_Hyst_BAM_F32.mdl');text(10,75,'Hysteresis function.');text(10,60,'NXP')
      | text(10,45,'0.1');text(10,30,'09-Apr-2014');
  logo : Subsystem
      mask Display: image(imread('logo.jpg'))
  f32Out : Outport
  wires:
  GFLIB_Hyst_SF_F32/1 -> f32Out/1
  f32In/1 -> GFLIB_Hyst_SF_F32/1
  Unit_Delay_f32InState/1 -> GFLIB_Hyst_SF_F32/2
  GFLIB_Hyst_SF_F32/2 -> Unit_Delay_f32InState/1

== system ammclib_bam_s32k14x/GFLIB/bam_f32/GFLIB_IntegratorTR_F32 ==
  note: ---------------------------------------------------------------------------------------------------------------------------------------------------------------------------------------------------
  f32In : Inport
  GFLIB_IntegratorTR_SF : S-Function  FunctionName=GFLIB_IntegratorTR_SF_F32  Parameters=f32C1,u16NShift  SFunctionDeploymentMode=off  EnableBusSupport=off
  Unit_Delay_f32InAcc : UnitDelay  SampleTime=-1
  Unit_Delay_f32InK_1 : UnitDelay  SampleTime=-1
  copyright : Subsystem
      mask Display:
      | text(10,90,'FILE:');text(10,75,'DESRIPTION:')
      | text(10,60,'COPYRIGHT:')
      | text(10,45,'VERSION:')
      | text(10,30,'DATE:')
  copyright2 : Subsystem
      mask Display:
      | text(10,90,'GFLIB_IntegratorTR_BAM_F32.mdl');text(10,75,'Discrete integrator transformed from linear model using Billinear (trapezoidal) transformation.');text(10,60,'NXP')
      | text(10,45,'0.1');text(10,30,'16-Jan-2012');
  logo : Subsystem
      mask Display: image(imread('logo.jpg'))
  f32Out : Outport
  wires:
  GFLIB_IntegratorTR_SF/1 -> f32Out/1
  f32In/1 -> GFLIB_IntegratorTR_SF/1
  GFLIB_IntegratorTR_SF/3 -> Unit_Delay_f32InK_1/1
  Unit_Delay_f32InK_1/1 -> GFLIB_IntegratorTR_SF/3
  Unit_Delay_f32InAcc/1 -> GFLIB_IntegratorTR_SF/2
  GFLIB_IntegratorTR_SF/2 -> Unit_Delay_f32InAcc/1

== system ammclib_bam_s32k14x/GFLIB/bam_f32/GFLIB_Limit_F32 ==
  note: ---------------------------------------------------------------------------------------------------------------------------------------------------------------------------------------------------
  f32In : Inport
  GFLIB_Limit_SF_F32 : S-Function  FunctionName=GFLIB_Limit_SF_F32  Parameters=f32UpperLimit,f32LowerLim  SFunctionDeploymentMode=off  EnableBusSupport=off
  copyright : Subsystem
      mask Display:
      | text(10,90,'FILE:');text(10,75,'DESRIPTION:')
      | text(10,60,'COPYRIGHT:')
      | text(10,45,'VERSION:')
      | text(10,30,'DATE:')
      | text(10,15,'AUTHOR:')
  copyright2 : Subsystem
      mask Display:
      | text(10,90,'GFLIB_Limit_BAM_F32.mdl');text(10,75,'Limit function');text(10,60,'NXP')
      | text(10,45,'0.1');text(10,30,'03-Jul-2011');text(10,15,'');
  logo : Subsystem
      mask Display: image(imread('logo.jpg'))
  f32Out : Outport
  wires:
  GFLIB_Limit_SF_F32/1 -> f32Out/1
  f32In/1 -> GFLIB_Limit_SF_F32/1

== system ammclib_bam_s32k14x/GFLIB/bam_f32/GFLIB_LowerLimit_F32 ==
  note: ---------------------------------------------------------------------------------------------------------------------------------------------------------------------------------------------------
  f32In : Inport
  GFLIB_LowerLimit_SF_F32 : S-Function  FunctionName=GFLIB_LowerLimit_SF_F32  Parameters=f32LowerLim  SFunctionDeploymentMode=off  EnableBusSupport=off
  copyright : Subsystem
      mask Display:
      | text(10,90,'FILE:');text(10,75,'DESRIPTION:')
      | text(10,60,'COPYRIGHT:')
      | text(10,45,'VERSION:')
      | text(10,30,'DATE:')
  copyright2 : Subsystem
      mask Display:
      | text(10,90,'GFLIB_LowerLimit_BAM_F32.mdl');text(10,75,'Lower limit function.');text(10,60,'Freescale')
      | text(10,45,'0.1');text(10,30,'13-Sep-2011');
  logo : Subsystem
      mask Display: image(imread('logo.jpg'))
  f32Out : Outport
  wires:
  GFLIB_LowerLimit_SF_F32/1 -> f32Out/1
  f32In/1 -> GFLIB_LowerLimit_SF_F32/1

== system ammclib_bam_s32k14x/GFLIB/bam_f32/GFLIB_Lut1D_F32 ==
  note: ---------------------------------------------------------------------------------------------------------------------------------------------------------------------------------------------------
  f32In : Inport
  GFLIB_Lut1D_SF : S-Function  FunctionName=GFLIB_Lut1D_SF_F32  Parameters=u32ShamOffset,pf32Table,s32MidIdx  SFunctionDeploymentMode=off  EnableBusSupport=off
  copyright : Subsystem
      mask Display:
      | text(10,90,'FILE:');text(10,75,'DESRIPTION:')
      | text(10,60,'COPYRIGHT:')
      | text(10,45,'VERSION:')
      | text(10,30,'DATE:')
  copyright2 : Subsystem
      mask Display:
      | text(10,90,'GFLIB_Lut1D_BAM_F32.mdl');text(10,75,'One dimensional Look-up table function');text(10,60,'NXP')
      | text(10,45,'0.1');text(10,30,'17-Jun-2013');
  logo : Subsystem
      mask Display: image(imread('logo.jpg'))
  f32Out : Outport
  wires:
  GFLIB_Lut1D_SF/1 -> f32Out/1
  f32In/1 -> GFLIB_Lut1D_SF/1

== system ammclib_bam_s32k14x/GFLIB/bam_f32/GFLIB_Lut2D_F32 ==
  note: ---------------------------------------------------------------------------------------------------------------------------------------------------------------------------------------------------
  f32In1 : Inport
  f32In2 : Inport  Port=2
  GFLIB_Lut2D_SF : S-Function  FunctionName=GFLIB_Lut2D_SF_F32  Parameters=u32ShamOffset1,u32ShamOffset2,pf32Table,s32MidIdx  SFunctionDeploymentMode=off  EnableBusSupport=off
  copyright : Subsystem
      mask Display:
      | text(10,90,'FILE:');text(10,75,'DESRIPTION:')
      | text(10,60,'COPYRIGHT:')
      | text(10,45,'VERSION:')
      | text(10,30,'DATE:')
  copyright2 : Subsystem
      mask Display:
      | text(10,90,'GFLIB_Lut2D_BAM_F32.mdl');text(10,75,'Two dimensional Look-up table function');text(10,60,'NXP')
      | text(10,45,'0.1');text(10,30,'17-Jun-2013');
  logo : Subsystem
      mask Display: image(imread('logo.jpg'))
  f32Out : Outport
  wires:
  GFLIB_Lut2D_SF/1 -> f32Out/1
  f32In2/1 -> GFLIB_Lut2D_SF/2
  f32In1/1 -> GFLIB_Lut2D_SF/1

== system ammclib_bam_s32k14x/GFLIB/bam_f32/GFLIB_Ramp_F32 ==
  note: ---------------------------------------------------------------------------------------------------------------------------------------------------------------------------------------------------
  f32In : Inport
  GFLIB_Ramp_SF_F32 : S-Function  FunctionName=GFLIB_Ramp_SF_F32  Parameters=f32RampUp,f32RampDown  SFunctionDeploymentMode=off  EnableBusSupport=off
  Unit_Delay_f32InState : UnitDelay  SampleTime=-1
  copyright : Subsystem
      mask Display:
      | text(10,90,'FILE:');text(10,75,'DESRIPTION:')
      | text(10,60,'COPYRIGHT:')
      | text(10,45,'VERSION:')
      | text(10,30,'DATE:')
      | text(10,15,'AUTHOR:')
  copyright2 : Subsystem
      mask Display:
      | text(10,90,'GFLIB_Ramp_BAM_F32.mdl');text(10,75,'Rate of change limiter - Ramp function.');text(10,60,'NXP')
      | text(10,45,'0.1');text(10,30,'08-Apr-2014');text(10,15,'');
  logo : Subsystem
      mask Display: image(imread('logo.jpg'))
  f32Out : Outport
  wires:
  GFLIB_Ramp_SF_F32/1 -> f32Out/1
  f32In/1 -> GFLIB_Ramp_SF_F32/1
  Unit_Delay_f32InState/1 -> GFLIB_Ramp_SF_F32/2
  GFLIB_Ramp_SF_F32/2 -> Unit_Delay_f32InState/1

== system ammclib_bam_s32k14x/GFLIB/bam_f32/GFLIB_Sign_F32 ==
  note: ---------------------------------------------------------------------------------------------------------------------------------------------------------------------------------------------------
  f32In : Inport
  GFLIB_Sign_SF_F32 : S-Function  FunctionName=GFLIB_Sign_SF_F32  SFunctionDeploymentMode=off  EnableBusSupport=off
  copyright : Subsystem
      mask Display:
      | text(10,90,'FILE:');text(10,75,'DESRIPTION:')
      | text(10,60,'COPYRIGHT:')
      | text(10,45,'VERSION:')
      | text(10,30,'DATE:')
  copyright2 : Subsystem
      mask Display:
      | text(10,90,'GFLIB_Sign_BAM_F32.mdl');text(10,75,'Sign function.');text(10,60,'NXP')
      | text(10,45,'0.1');text(10,30,'26-Aug-2011');
  logo : Subsystem
      mask Display: image(imread('logo.jpg'))
  f32Out : Outport
  wires:
  GFLIB_Sign_SF_F32/1 -> f32Out/1
  f32In/1 -> GFLIB_Sign_SF_F32/1

== system ammclib_bam_s32k14x/GFLIB/bam_f32/GFLIB_SinCos_F32 ==
  note: ---------------------------------------------------------------------------------------------------------------------------------------------------------------------------------------------------
  f32In : Inport
  GFLIB_SinCos_SF : S-Function  FunctionName=GFLIB_SinCos_SF_F32  SFunctionDeploymentMode=off  EnableBusSupport=off
  copyright : Subsystem
      mask Display: text(10,90,'FILE:');text(10,75,'DESRIPTION:');text(10,60,'COPYRIGHT:');text(10,45,'VERSION:');text(10,30,'DATE:')
  copyright2 : Subsystem
      mask Display: text(10,90,'GFLIB_SinCos_BAM_F32.mdl');text(10,75,'Sine and Cosine transformation');text(10,60,'Freescale');text(10,45,'0.1');text(10,30,'27-Sep-2015');
  logo : Subsystem
      mask Display: image(imread('logo.jpg'))
  f32SinOut : Outport
  f32CosOut : Outport  Port=2
  wires:
  GFLIB_SinCos_SF/2 -> f32CosOut/1
  GFLIB_SinCos_SF/1 -> f32SinOut/1
  f32In/1 -> GFLIB_SinCos_SF/1
